simulink model "scheme1"  (R2014a)
settings: Solver=ode3  StartTime=0.0  StopTime=0.05  FixedStep=1e-6  MaxStep=0.001  MinStep=0.0001  RelTol=1e-3
settings Model: Creator=User  LastModifiedBy=Анастасия

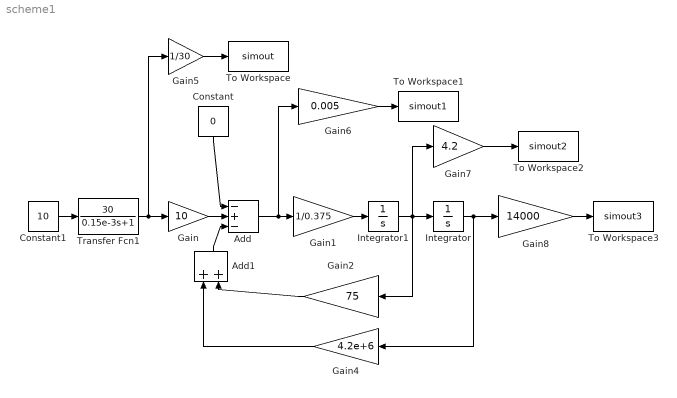
== system scheme1 ==
  Add : Sum  Inputs=-+-
  Add1 : Sum
  Constant : Constant  Value=0
  Constant1 : Constant  Value=10
  Gain : Gain  Gain=10
  Gain1 : Gain  Gain=1/0.375
  Gain2 : Gain  Gain=75
  Gain4 : Gain  Gain=4.2e+6
  Gain5 : Gain  Gain=1/30
  Gain6 : Gain  Gain=0.005
  Gain7 : Gain  Gain=4.2
  Gain8 : Gain  Gain=14000
  Integrator : Integrator
  Integrator1 : Integrator
  To Workspace : ToWorkspace  VariableName=simout  SaveFormat=Timeseries  SampleTime=-1
  To Workspace1 : ToWorkspace  VariableName=simout1  SaveFormat=Timeseries  SampleTime=-1
  To Workspace2 : ToWorkspace  VariableName=simout2  SaveFormat=Timeseries  SampleTime=-1
  To Workspace3 : ToWorkspace  VariableName=simout3  SaveFormat=Timeseries  SampleTime=-1
  Transfer Fcn1 : TransferFcn  Numerator=[30]  Denominator=[0.15e-3 1]
  wires:
  Constant1/1 -> Transfer Fcn1/1
  Transfer Fcn1/1 -> Gain/1, Gain5/1
  Integrator1/1 -> Integrator/1, Gain2/1, Gain7/1
  Integrator/1 -> Gain8/1, Gain4/1
  Gain8/1 -> To Workspace3/1
  Gain7/1 -> To Workspace2/1
  Gain6/1 -> To Workspace1/1
  Gain5/1 -> To Workspace/1
  Gain/1 -> Add/2
  Add1/1 -> Add/3
  Add/1 -> Gain6/1, Gain1/1
  Constant/1 -> Add/1
  Gain1/1 -> Integrator1/1
  Gain2/1 -> Add1/2
  Gain4/1 -> Add1/1
